simulink model "Sim2"  (R2023b)
settings: Solver=VariableStepAuto  StartTime=0.0  StopTime=50  RelTol=1e-3
values from neighbouring files (symbols this model uses):
  G = 0.000180    (= 0.00018)    [Simulador.m]    (also in Simulador2.m = 32.772667)
  K = 55555    [Simulador.m]    (also in Simulador2.m = 0.15)
  tau = 0.1    [Simulador.m]    (also in Simulador2.m)
  Ti = 0.1    [Simulador.m]    (also in Simulador2.m)
  TT = 0.9    [Simulador2.m]
settings Model: Creator=rodsc  LastModifiedBy=rodsc

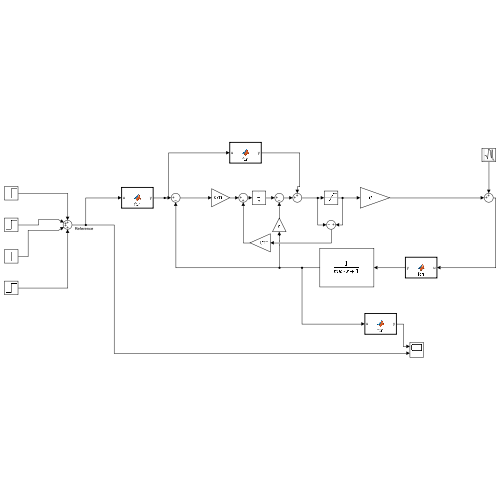
[thumbnail: Simulink's stored preview of the top-level diagram]
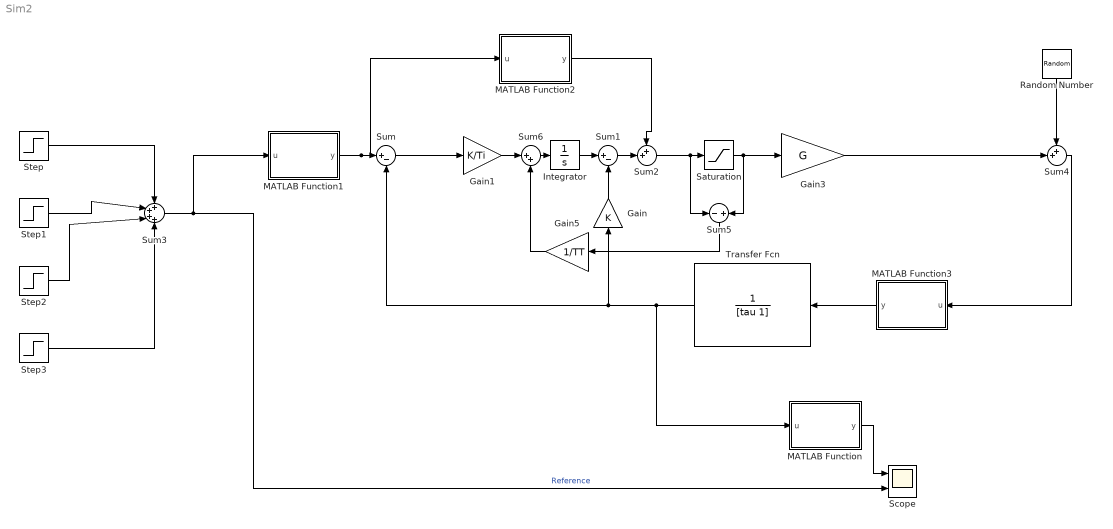
== system Sim2 ==
  Gain : Gain  Gain=K
  Gain1 : Gain  Gain=K/Ti
  Gain3 : Gain  Gain=G
  Gain5 : Gain  Gain=1/TT
  Integrator : Integrator
  MATLAB Function : MATLAB Function  TreatAsAtomicUnit=on
  MATLAB Function1 : MATLAB Function  TreatAsAtomicUnit=on
  MATLAB Function2 : MATLAB Function  TreatAsAtomicUnit=on
  MATLAB Function3 : MATLAB Function  TreatAsAtomicUnit=on
  Random Number : RandomNumber  Mean=0.28  Variance=0.001  SampleTime=0.1
  Saturation : Saturate  UpperLimit=1  LowerLimit=0
  Scope : Scope  NumInputPorts=2
  Step : Step  Time=4  After=10  SampleTime=0
  Step1 : Step  Time=15  After=15  SampleTime=0
  Step2 : Step  Time=30  After=-20  SampleTime=0
  Step3 : Step  Time=45  After=20  SampleTime=0
  Sum : Sum  Inputs=|+-
  Sum1 : Sum  Inputs=|+-
  Sum2 : Sum  Inputs=++|
  Sum3 : Sum  Inputs=++++
  Sum4 : Sum  Inputs=++|
  Sum5 : Sum  Inputs=-|+
  Sum6 : Sum  Inputs=|++
  Transfer Fcn : TransferFcn  Denominator=[tau 1]
  wires:
  Transfer Fcn/1 -> MATLAB Function/1(u), Gain/1, Sum/2
  Sum4/1 -> MATLAB Function3/1(u)
  MATLAB Function1/1(y) -> MATLAB Function2/1(u), Sum/1
  Gain/1 -> Sum1/2
  Sum1/1 -> Sum2/2
  Integrator/1 -> Sum1/1
  MATLAB Function2/1(y) -> Sum2/1
  Gain3/1 -> Sum4/2
  Step/1 -> Sum3/1
  Step1/1 -> Sum3/2
  Step2/1 -> Sum3/3
  Step3/1 -> Sum3/4
  Sum3/1 -> MATLAB Function1/1(u), Scope/2  "Reference"
  Random Number/1 -> Sum4/1
  Sum6/1 -> Integrator/1
  Gain1/1 -> Sum6/1
  Sum5/1 -> Gain5/1
  Gain5/1 -> Sum6/2
  Sum2/1 -> Sum5/1, Saturation/1
  Saturation/1 -> Gain3/1, Sum5/2
  Sum/1 -> Gain1/1
  MATLAB Function3/1(y) -> Transfer Fcn/1
  MATLAB Function/1(y) -> Scope/1

== matlab function Sim2/MATLAB Function2 ==
  data: u input; y output
function y = fcn(u)
%% Calcular H

%Volt to lux
if u~=0
G = 32.772667;
m = -0.89;
R1 = 10000.0;
VCC = 3.3;
offset_R_Lux = log10(225000) - m;
LDR_resistance = (VCC * R1) / u - R1;
lux = 10^((log10(LDR_resistance) - offset_R_Lux)/m);
H = u/lux;
%% Calcular b*K
y = u/(H*G);
else
    y = 0;
end

== matlab function Sim2/MATLAB Function3 ==
  data: u input; y output
function y = fcn(u)
m = -0.89;
R1 = 10000.0;
VCC = 3.3;
offset_R_Lux = log10(225000) - m;
resistance = 10^(m * log10(u) + offset_R_Lux);
y = (VCC * R1) / (resistance + R1);

== matlab function Sim2/MATLAB Function ==
  data: u input; y output
%Volt to lux

function y = fcn(u)
m = -0.89;
R1 = 10000.0;
VCC = 3.3;
offset_R_Lux = log10(225000) - m;
LDR_resistance = (VCC * R1) / u - R1;
y = 10^((log10(LDR_resistance) - offset_R_Lux)/m);

== matlab function Sim2/MATLAB Function1 ==
  data: u input; y output
function y = fcn(u)
m = -0.89;
R1 = 10000.0;
VCC = 3.3;
offset_R_Lux = log10(225000) - m;
resistance = 10^(m * log10(u) + offset_R_Lux);
y = (VCC * R1) / (resistance + R1);
